simulink model "mVeh_fun_tbm"  (R2023b)
settings: Solver=FixedStepDiscrete  StartTime=0.0  StopTime=Parm_cnv_simulink_stopTime  FixedStep=Const_cnv_fundmt_stepSize  RelTol=1e-3  EnableMultiTasking=on
InitFcn:
  | preLoadFun
undefined symbols (not defined in the file or in its folder): Calib_pirelle_presSnr_x8, Calib_roadTriger_x6, Calib_tbm_brkBts_x8, Calib_tbm_ctr_x8, Calib_tbm_sensor_x4, Calib_tbm_strDistb_x8, Calib_tbm_supCtr_x8, CtrSet_tbm_enab_x8, IO397, Parm_tbmVeh_sig_max_numInvalid, Parm_tbmVeh_sig_tolerate_numInvalid
libraries: canmsglib x34, speedgoatlib_IO691 x19, MyLibrary x5, libtb_gen_canMsgCntr x5, speedgoatlib_fpga_analog_io x1, simulink x1, speedgoatlib_fpga x1, lib_decmp_CtrSet_tbm_enab_x8 x1, lib_decmp_Calib_tbm_brkPreTriger_x6 x1, lib_decmp_Calib_tbm_sensor_x4 x1
(part 3 of 3)

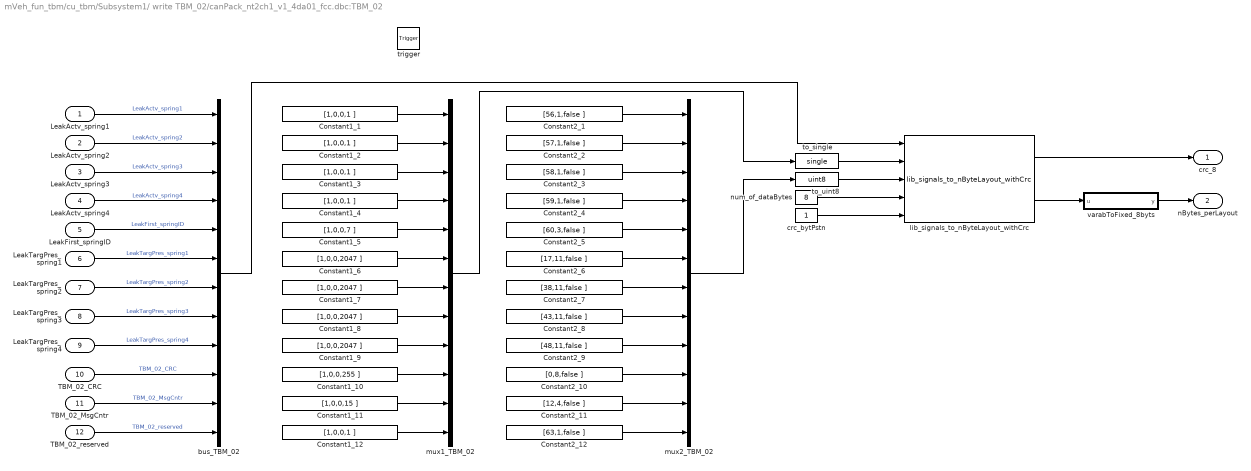
== system mVeh_fun_tbm/cu_tbm/Subsystem1/ write TBM_02/canPack_nt2ch1_v1_4da01_fcc.dbc:TBM_02 ==
  LeakActv_spring1 : Inport
  LeakActv_spring2 : Inport  Port=2
  LeakActv_spring3 : Inport  Port=3
  LeakActv_spring4 : Inport  Port=4
  LeakFirst_springID : Inport  Port=5
  LeakTargPres_spring1 : Inport  Port=6
  LeakTargPres_spring2 : Inport  Port=7
  LeakTargPres_spring3 : Inport  Port=8
  LeakTargPres_spring4 : Inport  Port=9
  TBM_02_CRC : Inport  Port=10
  TBM_02_MsgCntr : Inport  Port=11
  TBM_02_reserved : Inport  Port=12
  trigger : TriggerPort  TriggerType=either  VariantControl=Variant  PortDimensions=1
  Constant1_{1..4,12} (5 alike) : Constant  Value=[1,0,0,1 ]  SampleTime=-1
  Constant1_10 : Constant  Value=[1,0,0,255 ]  SampleTime=-1
  Constant1_11 : Constant  Value=[1,0,0,15 ]  SampleTime=-1
  Constant1_5 : Constant  Value=[1,0,0,7 ]  SampleTime=-1
  Constant1_{6..9} (4 alike) : Constant  Value=[1,0,0,2047 ]  SampleTime=-1
  Constant2_1 : Constant  Value=[56,1,false ]  SampleTime=-1
  Constant2_10 : Constant  Value=[0,8,false ]  SampleTime=-1
  Constant2_11 : Constant  Value=[12,4,false ]  SampleTime=-1
  Constant2_12 : Constant  Value=[63,1,false ]  SampleTime=-1
  Constant2_2 : Constant  Value=[57,1,false ]  SampleTime=-1
  Constant2_3 : Constant  Value=[58,1,false ]  SampleTime=-1
  Constant2_4 : Constant  Value=[59,1,false ]  SampleTime=-1
  Constant2_5 : Constant  Value=[60,3,false ]  SampleTime=-1
  Constant2_6 : Constant  Value=[17,11,false ]  SampleTime=-1
  Constant2_7 : Constant  Value=[38,11,false ]  SampleTime=-1
  Constant2_8 : Constant  Value=[43,11,false ]  SampleTime=-1
  Constant2_9 : Constant  Value=[48,11,false ]  SampleTime=-1
  bus_TBM_02 : BusCreator  Inputs=12
  crc_bytPstn : Constant  OutDataTypeStr=uint8  SampleTime=-1
  lib_signals_to_nByteLayout_withCrc : MyLibrary/lib_signals_to_nByteLayout_withCrc  SystemSampleTime=-1  VariantActivationTime=update diagram  AllowFlexibleInterface=on  Latency=0  AutoFrameSizeCalculation=off
  mux1_TBM_02 : Mux  Inputs=12
  mux2_TBM_02 : Mux  Inputs=12
  num_of_dataBytes : Constant  Value=8  OutDataTypeStr=uint8  SampleTime=-1
  to_single : DataTypeConversion  OutDataTypeStr=single  SaturateOnIntegerOverflow=off  RndMeth=Floor
  to_uint8 : DataTypeConversion  OutDataTypeStr=uint8  SaturateOnIntegerOverflow=off  RndMeth=Floor
  varabToFixed_8byts : MATLAB Function  TreatAsAtomicUnit=on
  crc_8 : Outport
  nBytes_perLayout : Outport  Port=2
  wires:
  LeakActv_spring1/1 -> bus_TBM_02/1  "LeakActv_spring1"
  LeakActv_spring2/1 -> bus_TBM_02/2  "LeakActv_spring2"
  LeakActv_spring3/1 -> bus_TBM_02/3  "LeakActv_spring3"
  LeakActv_spring4/1 -> bus_TBM_02/4  "LeakActv_spring4"
  LeakFirst_springID/1 -> bus_TBM_02/5  "LeakFirst_springID"
  LeakTargPres_spring1/1 -> bus_TBM_02/6  "LeakTargPres_spring1"
  LeakTargPres_spring2/1 -> bus_TBM_02/7  "LeakTargPres_spring2"
  LeakTargPres_spring3/1 -> bus_TBM_02/8  "LeakTargPres_spring3"
  LeakTargPres_spring4/1 -> bus_TBM_02/9  "LeakTargPres_spring4"
  TBM_02_CRC/1 -> bus_TBM_02/10  "TBM_02_CRC"
  TBM_02_MsgCntr/1 -> bus_TBM_02/11  "TBM_02_MsgCntr"
  TBM_02_reserved/1 -> bus_TBM_02/12  "TBM_02_reserved"
  Constant1_1/1 -> mux1_TBM_02/1
  Constant2_1/1 -> mux2_TBM_02/1
  Constant1_2/1 -> mux1_TBM_02/2
  Constant2_2/1 -> mux2_TBM_02/2
  Constant1_3/1 -> mux1_TBM_02/3
  Constant2_3/1 -> mux2_TBM_02/3
  Constant1_4/1 -> mux1_TBM_02/4
  Constant2_4/1 -> mux2_TBM_02/4
  Constant1_5/1 -> mux1_TBM_02/5
  Constant2_5/1 -> mux2_TBM_02/5
  Constant1_6/1 -> mux1_TBM_02/6
  Constant2_6/1 -> mux2_TBM_02/6
  Constant1_7/1 -> mux1_TBM_02/7
  Constant2_7/1 -> mux2_TBM_02/7
  Constant1_8/1 -> mux1_TBM_02/8
  Constant2_8/1 -> mux2_TBM_02/8
  Constant1_9/1 -> mux1_TBM_02/9
  Constant2_9/1 -> mux2_TBM_02/9
  Constant1_10/1 -> mux1_TBM_02/10
  Constant2_10/1 -> mux2_TBM_02/10
  Constant1_11/1 -> mux1_TBM_02/11
  Constant2_11/1 -> mux2_TBM_02/11
  Constant1_12/1 -> mux1_TBM_02/12
  Constant2_12/1 -> mux2_TBM_02/12
  bus_TBM_02/1 -> lib_signals_to_nByteLayout_withCrc/1
  mux1_TBM_02/1 -> to_single/1
  to_single/1 -> lib_signals_to_nByteLayout_withCrc/2
  mux2_TBM_02/1 -> to_uint8/1
  to_uint8/1 -> lib_signals_to_nByteLayout_withCrc/3
  lib_signals_to_nByteLayout_withCrc/1 -> crc_8/1
  num_of_dataBytes/1 -> lib_signals_to_nByteLayout_withCrc/4
  lib_signals_to_nByteLayout_withCrc/2 -> varabToFixed_8byts/1(u)
  varabToFixed_8byts/1(y) -> nBytes_perLayout/1
  crc_bytPstn/1 -> lib_signals_to_nByteLayout_withCrc/5

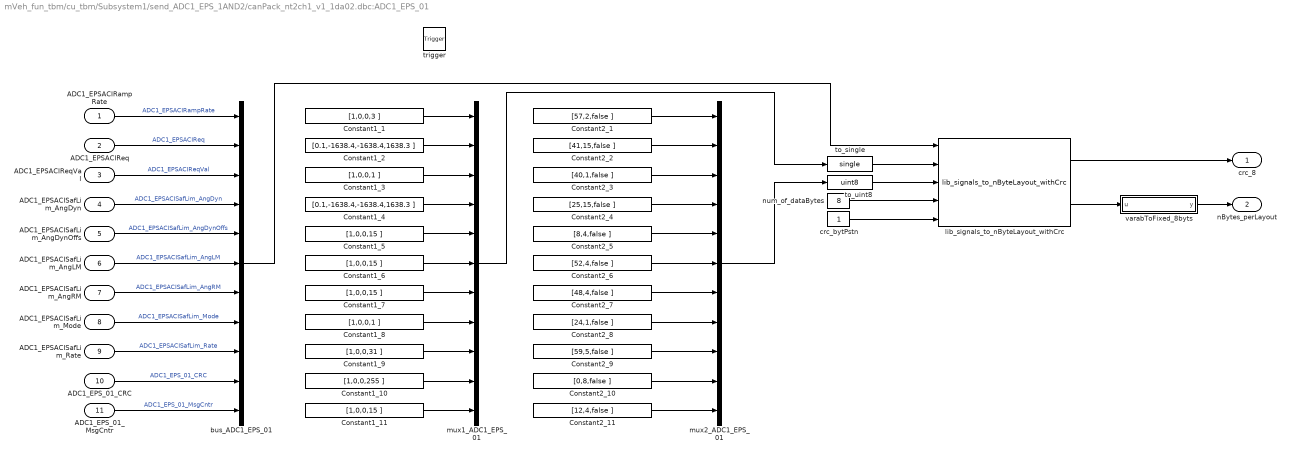
== system mVeh_fun_tbm/cu_tbm/Subsystem1/send_ADC1_EPS_1AND2/canPack_nt2ch1_v1_1da02.dbc:ADC1_EPS_01 ==
  ADC1_EPSACIRampRate : Inport
  ADC1_EPSACIReq : Inport  Port=2
  ADC1_EPSACIReqVal : Inport  Port=3
  ADC1_EPSACISafLim_AngDyn : Inport  Port=4
  ADC1_EPSACISafLim_AngDynOffs : Inport  Port=5
  ADC1_EPSACISafLim_AngLM : Inport  Port=6
  ADC1_EPSACISafLim_AngRM : Inport  Port=7
  ADC1_EPSACISafLim_Mode : Inport  Port=8
  ADC1_EPSACISafLim_Rate : Inport  Port=9
  ADC1_EPS_01_CRC : Inport  Port=10
  ADC1_EPS_01_MsgCntr : Inport  Port=11
  trigger : TriggerPort  TriggerType=either  VariantControl=Variant  PortDimensions=1
  Constant1_1 : Constant  Value=[1,0,0,3 ]  SampleTime=-1
  Constant1_10 : Constant  Value=[1,0,0,255 ]  SampleTime=-1
  Constant1_{5..7,11} (4 alike) : Constant  Value=[1,0,0,15 ]  SampleTime=-1
  Constant1_2 : Constant  Value=[0.1,-1638.4,-1638.4,1638.3 ]  SampleTime=-1
  Constant1_3 : Constant  Value=[1,0,0,1 ]  SampleTime=-1
  Constant1_4 : Constant  Value=[0.1,-1638.4,-1638.4,1638.3 ]  SampleTime=-1
  Constant1_8 : Constant  Value=[1,0,0,1 ]  SampleTime=-1
  Constant1_9 : Constant  Value=[1,0,0,31 ]  SampleTime=-1
  Constant2_1 : Constant  Value=[57,2,false ]  SampleTime=-1
  Constant2_10 : Constant  Value=[0,8,false ]  SampleTime=-1
  Constant2_11 : Constant  Value=[12,4,false ]  SampleTime=-1
  Constant2_2 : Constant  Value=[41,15,false ]  SampleTime=-1
  Constant2_3 : Constant  Value=[40,1,false ]  SampleTime=-1
  Constant2_4 : Constant  Value=[25,15,false ]  SampleTime=-1
  Constant2_5 : Constant  Value=[8,4,false ]  SampleTime=-1
  Constant2_6 : Constant  Value=[52,4,false ]  SampleTime=-1
  Constant2_7 : Constant  Value=[48,4,false ]  SampleTime=-1
  Constant2_8 : Constant  Value=[24,1,false ]  SampleTime=-1
  Constant2_9 : Constant  Value=[59,5,false ]  SampleTime=-1
  bus_ADC1_EPS_01 : BusCreator  Inputs=11
  crc_bytPstn : Constant  OutDataTypeStr=uint8  SampleTime=-1
  lib_signals_to_nByteLayout_withCrc : MyLibrary/lib_signals_to_nByteLayout_withCrc  SystemSampleTime=-1  VariantActivationTime=update diagram  AllowFlexibleInterface=on  Latency=0  AutoFrameSizeCalculation=off
  mux1_ADC1_EPS_01 : Mux  Inputs=11
  mux2_ADC1_EPS_01 : Mux  Inputs=11
  num_of_dataBytes : Constant  Value=8  OutDataTypeStr=uint8  SampleTime=-1
  to_single : DataTypeConversion  OutDataTypeStr=single  SaturateOnIntegerOverflow=off  RndMeth=Floor
  to_uint8 : DataTypeConversion  OutDataTypeStr=uint8  SaturateOnIntegerOverflow=off  RndMeth=Floor
  varabToFixed_8byts : MATLAB Function  TreatAsAtomicUnit=on
  crc_8 : Outport
  nBytes_perLayout : Outport  Port=2
  wires:
  ADC1_EPSACIRampRate/1 -> bus_ADC1_EPS_01/1  "ADC1_EPSACIRampRate"
  ADC1_EPSACIReq/1 -> bus_ADC1_EPS_01/2  "ADC1_EPSACIReq"
  ADC1_EPSACIReqVal/1 -> bus_ADC1_EPS_01/3  "ADC1_EPSACIReqVal"
  ADC1_EPSACISafLim_AngDyn/1 -> bus_ADC1_EPS_01/4  "ADC1_EPSACISafLim_AngDyn"
  ADC1_EPSACISafLim_AngDynOffs/1 -> bus_ADC1_EPS_01/5  "ADC1_EPSACISafLim_AngDynOffs"
  ADC1_EPSACISafLim_AngLM/1 -> bus_ADC1_EPS_01/6  "ADC1_EPSACISafLim_AngLM"
  ADC1_EPSACISafLim_AngRM/1 -> bus_ADC1_EPS_01/7  "ADC1_EPSACISafLim_AngRM"
  ADC1_EPSACISafLim_Mode/1 -> bus_ADC1_EPS_01/8  "ADC1_EPSACISafLim_Mode"
  ADC1_EPSACISafLim_Rate/1 -> bus_ADC1_EPS_01/9  "ADC1_EPSACISafLim_Rate"
  ADC1_EPS_01_CRC/1 -> bus_ADC1_EPS_01/10  "ADC1_EPS_01_CRC"
  ADC1_EPS_01_MsgCntr/1 -> bus_ADC1_EPS_01/11  "ADC1_EPS_01_MsgCntr"
  Constant1_1/1 -> mux1_ADC1_EPS_01/1
  Constant2_1/1 -> mux2_ADC1_EPS_01/1
  Constant1_2/1 -> mux1_ADC1_EPS_01/2
  Constant2_2/1 -> mux2_ADC1_EPS_01/2
  Constant1_3/1 -> mux1_ADC1_EPS_01/3
  Constant2_3/1 -> mux2_ADC1_EPS_01/3
  Constant1_4/1 -> mux1_ADC1_EPS_01/4
  Constant2_4/1 -> mux2_ADC1_EPS_01/4
  Constant1_5/1 -> mux1_ADC1_EPS_01/5
  Constant2_5/1 -> mux2_ADC1_EPS_01/5
  Constant1_6/1 -> mux1_ADC1_EPS_01/6
  Constant2_6/1 -> mux2_ADC1_EPS_01/6
  Constant1_7/1 -> mux1_ADC1_EPS_01/7
  Constant2_7/1 -> mux2_ADC1_EPS_01/7
  Constant1_8/1 -> mux1_ADC1_EPS_01/8
  Constant2_8/1 -> mux2_ADC1_EPS_01/8
  Constant1_9/1 -> mux1_ADC1_EPS_01/9
  Constant2_9/1 -> mux2_ADC1_EPS_01/9
  Constant1_10/1 -> mux1_ADC1_EPS_01/10
  Constant2_10/1 -> mux2_ADC1_EPS_01/10
  Constant1_11/1 -> mux1_ADC1_EPS_01/11
  Constant2_11/1 -> mux2_ADC1_EPS_01/11
  bus_ADC1_EPS_01/1 -> lib_signals_to_nByteLayout_withCrc/1
  mux1_ADC1_EPS_01/1 -> to_single/1
  to_single/1 -> lib_signals_to_nByteLayout_withCrc/2
  mux2_ADC1_EPS_01/1 -> to_uint8/1
  to_uint8/1 -> lib_signals_to_nByteLayout_withCrc/3
  lib_signals_to_nByteLayout_withCrc/1 -> crc_8/1
  num_of_dataBytes/1 -> lib_signals_to_nByteLayout_withCrc/4
  lib_signals_to_nByteLayout_withCrc/2 -> varabToFixed_8byts/1(u)
  varabToFixed_8byts/1(y) -> nBytes_perLayout/1
  crc_bytPstn/1 -> lib_signals_to_nByteLayout_withCrc/5

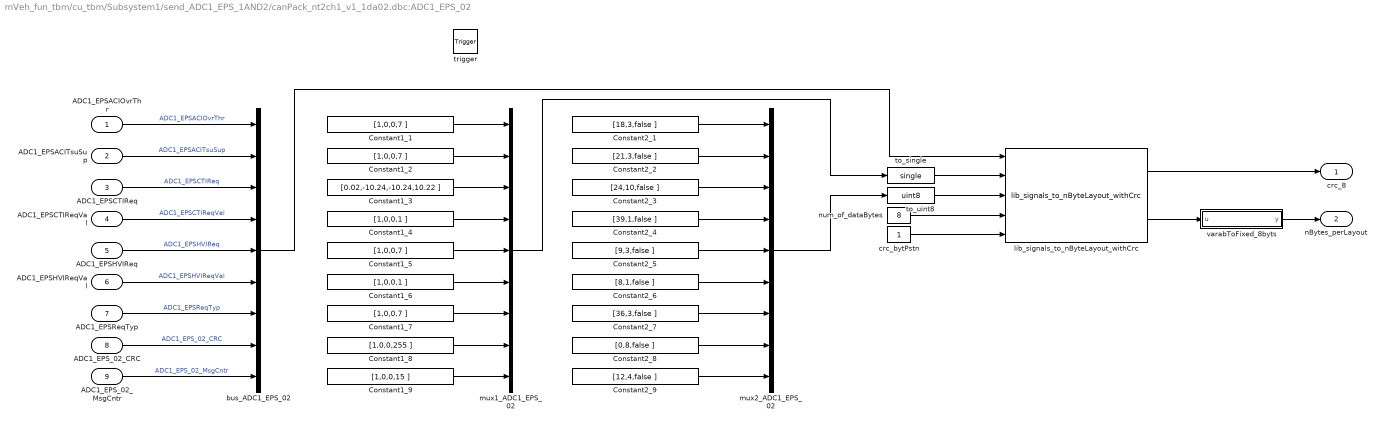
== system mVeh_fun_tbm/cu_tbm/Subsystem1/send_ADC1_EPS_1AND2/canPack_nt2ch1_v1_1da02.dbc:ADC1_EPS_02 ==
  ADC1_EPSACIOvrThr : Inport
  ADC1_EPSACITsuSup : Inport  Port=2
  ADC1_EPSCTIReq : Inport  Port=3
  ADC1_EPSCTIReqVal : Inport  Port=4
  ADC1_EPSHVIReq : Inport  Port=5
  ADC1_EPSHVIReqVal : Inport  Port=6
  ADC1_EPSReqTyp : Inport  Port=7
  ADC1_EPS_02_CRC : Inport  Port=8
  ADC1_EPS_02_MsgCntr : Inport  Port=9
  trigger : TriggerPort  TriggerType=either  VariantControl=Variant  PortDimensions=1
  Constant1_{1..2,5,7} (4 alike) : Constant  Value=[1,0,0,7 ]  SampleTime=-1
  Constant1_3 : Constant  Value=[0.02,-10.24,-10.24,10.22 ]  SampleTime=-1
  Constant1_4 : Constant  Value=[1,0,0,1 ]  SampleTime=-1
  Constant1_6 : Constant  Value=[1,0,0,1 ]  SampleTime=-1
  Constant1_8 : Constant  Value=[1,0,0,255 ]  SampleTime=-1
  Constant1_9 : Constant  Value=[1,0,0,15 ]  SampleTime=-1
  Constant2_1 : Constant  Value=[18,3,false ]  SampleTime=-1
  Constant2_2 : Constant  Value=[21,3,false ]  SampleTime=-1
  Constant2_3 : Constant  Value=[24,10,false ]  SampleTime=-1
  Constant2_4 : Constant  Value=[39,1,false ]  SampleTime=-1
  Constant2_5 : Constant  Value=[9,3,false ]  SampleTime=-1
  Constant2_6 : Constant  Value=[8,1,false ]  SampleTime=-1
  Constant2_7 : Constant  Value=[36,3,false ]  SampleTime=-1
  Constant2_8 : Constant  Value=[0,8,false ]  SampleTime=-1
  Constant2_9 : Constant  Value=[12,4,false ]  SampleTime=-1
  bus_ADC1_EPS_02 : BusCreator  Inputs=9
  crc_bytPstn : Constant  OutDataTypeStr=uint8  SampleTime=-1
  lib_signals_to_nByteLayout_withCrc : MyLibrary/lib_signals_to_nByteLayout_withCrc  SystemSampleTime=-1  VariantActivationTime=update diagram  AllowFlexibleInterface=on  Latency=0  AutoFrameSizeCalculation=off
  mux1_ADC1_EPS_02 : Mux  Inputs=9
  mux2_ADC1_EPS_02 : Mux  Inputs=9
  num_of_dataBytes : Constant  Value=8  OutDataTypeStr=uint8  SampleTime=-1
  to_single : DataTypeConversion  OutDataTypeStr=single  SaturateOnIntegerOverflow=off  RndMeth=Floor
  to_uint8 : DataTypeConversion  OutDataTypeStr=uint8  SaturateOnIntegerOverflow=off  RndMeth=Floor
  varabToFixed_8byts : MATLAB Function  TreatAsAtomicUnit=on
  crc_8 : Outport
  nBytes_perLayout : Outport  Port=2
  wires:
  ADC1_EPSACIOvrThr/1 -> bus_ADC1_EPS_02/1  "ADC1_EPSACIOvrThr"
  ADC1_EPSACITsuSup/1 -> bus_ADC1_EPS_02/2  "ADC1_EPSACITsuSup"
  ADC1_EPSCTIReq/1 -> bus_ADC1_EPS_02/3  "ADC1_EPSCTIReq"
  ADC1_EPSCTIReqVal/1 -> bus_ADC1_EPS_02/4  "ADC1_EPSCTIReqVal"
  ADC1_EPSHVIReq/1 -> bus_ADC1_EPS_02/5  "ADC1_EPSHVIReq"
  ADC1_EPSHVIReqVal/1 -> bus_ADC1_EPS_02/6  "ADC1_EPSHVIReqVal"
  ADC1_EPSReqTyp/1 -> bus_ADC1_EPS_02/7  "ADC1_EPSReqTyp"
  ADC1_EPS_02_CRC/1 -> bus_ADC1_EPS_02/8  "ADC1_EPS_02_CRC"
  ADC1_EPS_02_MsgCntr/1 -> bus_ADC1_EPS_02/9  "ADC1_EPS_02_MsgCntr"
  Constant1_1/1 -> mux1_ADC1_EPS_02/1
  Constant2_1/1 -> mux2_ADC1_EPS_02/1
  Constant1_2/1 -> mux1_ADC1_EPS_02/2
  Constant2_2/1 -> mux2_ADC1_EPS_02/2
  Constant1_3/1 -> mux1_ADC1_EPS_02/3
  Constant2_3/1 -> mux2_ADC1_EPS_02/3
  Constant1_4/1 -> mux1_ADC1_EPS_02/4
  Constant2_4/1 -> mux2_ADC1_EPS_02/4
  Constant1_5/1 -> mux1_ADC1_EPS_02/5
  Constant2_5/1 -> mux2_ADC1_EPS_02/5
  Constant1_6/1 -> mux1_ADC1_EPS_02/6
  Constant2_6/1 -> mux2_ADC1_EPS_02/6
  Constant1_7/1 -> mux1_ADC1_EPS_02/7
  Constant2_7/1 -> mux2_ADC1_EPS_02/7
  Constant1_8/1 -> mux1_ADC1_EPS_02/8
  Constant2_8/1 -> mux2_ADC1_EPS_02/8
  Constant1_9/1 -> mux1_ADC1_EPS_02/9
  Constant2_9/1 -> mux2_ADC1_EPS_02/9
  bus_ADC1_EPS_02/1 -> lib_signals_to_nByteLayout_withCrc/1
  mux1_ADC1_EPS_02/1 -> to_single/1
  to_single/1 -> lib_signals_to_nByteLayout_withCrc/2
  mux2_ADC1_EPS_02/1 -> to_uint8/1
  to_uint8/1 -> lib_signals_to_nByteLayout_withCrc/3
  lib_signals_to_nByteLayout_withCrc/1 -> crc_8/1
  num_of_dataBytes/1 -> lib_signals_to_nByteLayout_withCrc/4
  lib_signals_to_nByteLayout_withCrc/2 -> varabToFixed_8byts/1(u)
  varabToFixed_8byts/1(y) -> nBytes_perLayout/1
  crc_bytPstn/1 -> lib_signals_to_nByteLayout_withCrc/5

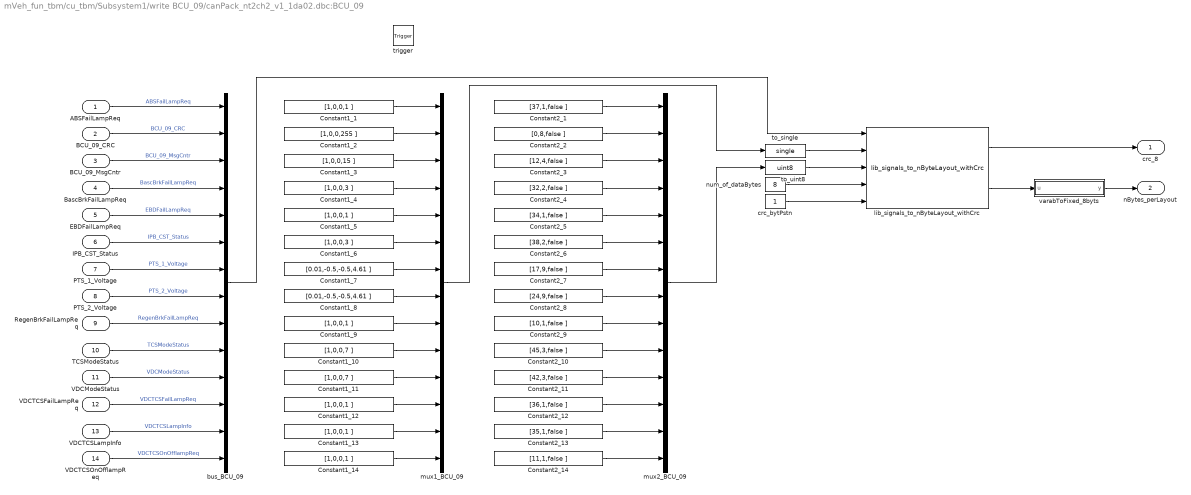
== system mVeh_fun_tbm/cu_tbm/Subsystem1/write BCU_09/canPack_nt2ch2_v1_1da02.dbc:BCU_09 ==
  ABSFailLampReq : Inport
  BCU_09_CRC : Inport  Port=2
  BCU_09_MsgCntr : Inport  Port=3
  BascBrkFailLampReq : Inport  Port=4
  EBDFailLampReq : Inport  Port=5
  IPB_CST_Status : Inport  Port=6
  PTS_1_Voltage : Inport  Port=7
  PTS_2_Voltage : Inport  Port=8
  RegenBrkFailLampReq : Inport  Port=9
  TCSModeStatus : Inport  Port=10
  VDCModeStatus : Inport  Port=11
  VDCTCSFailLampReq : Inport  Port=12
  VDCTCSLampInfo : Inport  Port=13
  VDCTCSOnOfflampReq : Inport  Port=14
  trigger : TriggerPort  TriggerType=either  VariantControl=Variant  PortDimensions=1
  Constant1_{1,5,9,12..14} (6 alike) : Constant  Value=[1,0,0,1 ]  SampleTime=-1
  Constant1_10 : Constant  Value=[1,0,0,7 ]  SampleTime=-1
  Constant1_11 : Constant  Value=[1,0,0,7 ]  SampleTime=-1
  Constant1_2 : Constant  Value=[1,0,0,255 ]  SampleTime=-1
  Constant1_3 : Constant  Value=[1,0,0,15 ]  SampleTime=-1
  Constant1_4 : Constant  Value=[1,0,0,3 ]  SampleTime=-1
  Constant1_6 : Constant  Value=[1,0,0,3 ]  SampleTime=-1
  Constant1_7 : Constant  Value=[0.01,-0.5,-0.5,4.61 ]  SampleTime=-1
  Constant1_8 : Constant  Value=[0.01,-0.5,-0.5,4.61 ]  SampleTime=-1
  Constant2_1 : Constant  Value=[37,1,false ]  SampleTime=-1
  Constant2_10 : Constant  Value=[45,3,false ]  SampleTime=-1
  Constant2_11 : Constant  Value=[42,3,false ]  SampleTime=-1
  Constant2_12 : Constant  Value=[36,1,false ]  SampleTime=-1
  Constant2_13 : Constant  Value=[35,1,false ]  SampleTime=-1
  Constant2_14 : Constant  Value=[11,1,false ]  SampleTime=-1
  Constant2_2 : Constant  Value=[0,8,false ]  SampleTime=-1
  Constant2_3 : Constant  Value=[12,4,false ]  SampleTime=-1
  Constant2_4 : Constant  Value=[32,2,false ]  SampleTime=-1
  Constant2_5 : Constant  Value=[34,1,false ]  SampleTime=-1
  Constant2_6 : Constant  Value=[38,2,false ]  SampleTime=-1
  Constant2_7 : Constant  Value=[17,9,false ]  SampleTime=-1
  Constant2_8 : Constant  Value=[24,9,false ]  SampleTime=-1
  Constant2_9 : Constant  Value=[10,1,false ]  SampleTime=-1
  bus_BCU_09 : BusCreator  Inputs=14
  crc_bytPstn : Constant  OutDataTypeStr=uint8  SampleTime=-1
  lib_signals_to_nByteLayout_withCrc : MyLibrary/lib_signals_to_nByteLayout_withCrc  SystemSampleTime=-1  VariantActivationTime=update diagram  AllowFlexibleInterface=on  Latency=0  AutoFrameSizeCalculation=off
  mux1_BCU_09 : Mux  Inputs=14
  mux2_BCU_09 : Mux  Inputs=14
  num_of_dataBytes : Constant  Value=8  OutDataTypeStr=uint8  SampleTime=-1
  to_single : DataTypeConversion  OutDataTypeStr=single  SaturateOnIntegerOverflow=off  RndMeth=Floor
  to_uint8 : DataTypeConversion  OutDataTypeStr=uint8  SaturateOnIntegerOverflow=off  RndMeth=Floor
  varabToFixed_8byts : MATLAB Function  TreatAsAtomicUnit=on
  crc_8 : Outport
  nBytes_perLayout : Outport  Port=2
  wires:
  ABSFailLampReq/1 -> bus_BCU_09/1  "ABSFailLampReq"
  BCU_09_CRC/1 -> bus_BCU_09/2  "BCU_09_CRC"
  BCU_09_MsgCntr/1 -> bus_BCU_09/3  "BCU_09_MsgCntr"
  BascBrkFailLampReq/1 -> bus_BCU_09/4  "BascBrkFailLampReq"
  EBDFailLampReq/1 -> bus_BCU_09/5  "EBDFailLampReq"
  IPB_CST_Status/1 -> bus_BCU_09/6  "IPB_CST_Status"
  PTS_1_Voltage/1 -> bus_BCU_09/7  "PTS_1_Voltage"
  PTS_2_Voltage/1 -> bus_BCU_09/8  "PTS_2_Voltage"
  RegenBrkFailLampReq/1 -> bus_BCU_09/9  "RegenBrkFailLampReq"
  TCSModeStatus/1 -> bus_BCU_09/10  "TCSModeStatus"
  VDCModeStatus/1 -> bus_BCU_09/11  "VDCModeStatus"
  VDCTCSFailLampReq/1 -> bus_BCU_09/12  "VDCTCSFailLampReq"
  VDCTCSLampInfo/1 -> bus_BCU_09/13  "VDCTCSLampInfo"
  VDCTCSOnOfflampReq/1 -> bus_BCU_09/14  "VDCTCSOnOfflampReq"
  Constant1_1/1 -> mux1_BCU_09/1
  Constant2_1/1 -> mux2_BCU_09/1
  Constant1_2/1 -> mux1_BCU_09/2
  Constant2_2/1 -> mux2_BCU_09/2
  Constant1_3/1 -> mux1_BCU_09/3
  Constant2_3/1 -> mux2_BCU_09/3
  Constant1_4/1 -> mux1_BCU_09/4
  Constant2_4/1 -> mux2_BCU_09/4
  Constant1_5/1 -> mux1_BCU_09/5
  Constant2_5/1 -> mux2_BCU_09/5
  Constant1_6/1 -> mux1_BCU_09/6
  Constant2_6/1 -> mux2_BCU_09/6
  Constant1_7/1 -> mux1_BCU_09/7
  Constant2_7/1 -> mux2_BCU_09/7
  Constant1_8/1 -> mux1_BCU_09/8
  Constant2_8/1 -> mux2_BCU_09/8
  Constant1_9/1 -> mux1_BCU_09/9
  Constant2_9/1 -> mux2_BCU_09/9
  Constant1_10/1 -> mux1_BCU_09/10
  Constant2_10/1 -> mux2_BCU_09/10
  Constant1_11/1 -> mux1_BCU_09/11
  Constant2_11/1 -> mux2_BCU_09/11
  Constant1_12/1 -> mux1_BCU_09/12
  Constant2_12/1 -> mux2_BCU_09/12
  Constant1_13/1 -> mux1_BCU_09/13
  Constant2_13/1 -> mux2_BCU_09/13
  Constant1_14/1 -> mux1_BCU_09/14
  Constant2_14/1 -> mux2_BCU_09/14
  bus_BCU_09/1 -> lib_signals_to_nByteLayout_withCrc/1
  mux1_BCU_09/1 -> to_single/1
  to_single/1 -> lib_signals_to_nByteLayout_withCrc/2
  mux2_BCU_09/1 -> to_uint8/1
  to_uint8/1 -> lib_signals_to_nByteLayout_withCrc/3
  lib_signals_to_nByteLayout_withCrc/1 -> crc_8/1
  num_of_dataBytes/1 -> lib_signals_to_nByteLayout_withCrc/4
  lib_signals_to_nByteLayout_withCrc/2 -> varabToFixed_8byts/1(u)
  varabToFixed_8byts/1(y) -> nBytes_perLayout/1
  crc_bytPstn/1 -> lib_signals_to_nByteLayout_withCrc/5

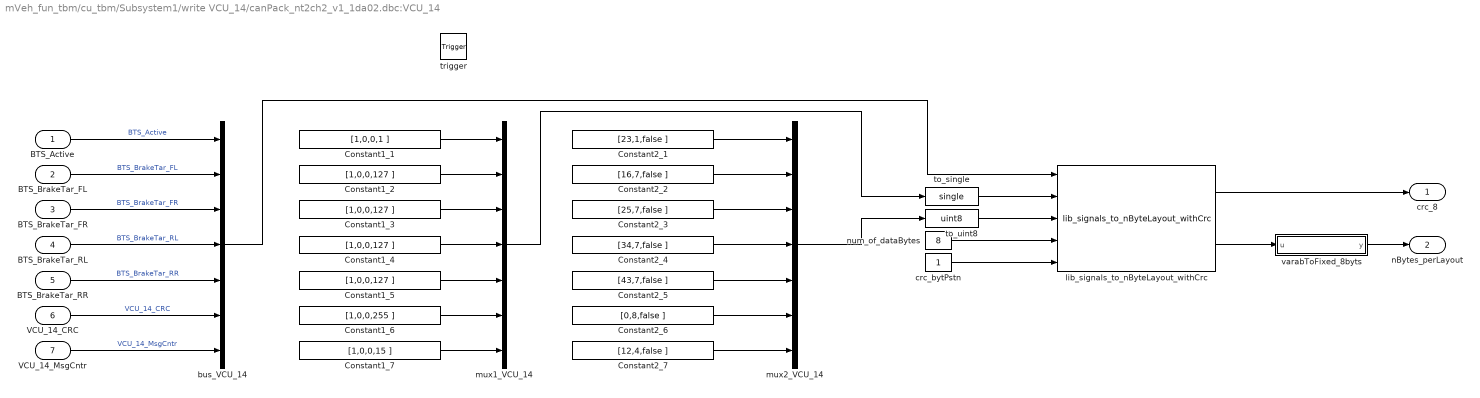
== system mVeh_fun_tbm/cu_tbm/Subsystem1/write VCU_14/canPack_nt2ch2_v1_1da02.dbc:VCU_14 ==
  BTS_Active : Inport
  BTS_BrakeTar_FL : Inport  Port=2
  BTS_BrakeTar_FR : Inport  Port=3
  BTS_BrakeTar_RL : Inport  Port=4
  BTS_BrakeTar_RR : Inport  Port=5
  VCU_14_CRC : Inport  Port=6
  VCU_14_MsgCntr : Inport  Port=7
  trigger : TriggerPort  TriggerType=either  VariantControl=Variant  PortDimensions=1
  Constant1_1 : Constant  Value=[1,0,0,1 ]  SampleTime=-1
  Constant1_{2..5} (4 alike) : Constant  Value=[1,0,0,127 ]  SampleTime=-1
  Constant1_6 : Constant  Value=[1,0,0,255 ]  SampleTime=-1
  Constant1_7 : Constant  Value=[1,0,0,15 ]  SampleTime=-1
  Constant2_1 : Constant  Value=[23,1,false ]  SampleTime=-1
  Constant2_2 : Constant  Value=[16,7,false ]  SampleTime=-1
  Constant2_3 : Constant  Value=[25,7,false ]  SampleTime=-1
  Constant2_4 : Constant  Value=[34,7,false ]  SampleTime=-1
  Constant2_5 : Constant  Value=[43,7,false ]  SampleTime=-1
  Constant2_6 : Constant  Value=[0,8,false ]  SampleTime=-1
  Constant2_7 : Constant  Value=[12,4,false ]  SampleTime=-1
  bus_VCU_14 : BusCreator  Inputs=7
  crc_bytPstn : Constant  OutDataTypeStr=uint8  SampleTime=-1
  lib_signals_to_nByteLayout_withCrc : MyLibrary/lib_signals_to_nByteLayout_withCrc  SystemSampleTime=-1  VariantActivationTime=update diagram  AllowFlexibleInterface=on  Latency=0  AutoFrameSizeCalculation=off
  mux1_VCU_14 : Mux  Inputs=7
  mux2_VCU_14 : Mux  Inputs=7
  num_of_dataBytes : Constant  Value=8  OutDataTypeStr=uint8  SampleTime=-1
  to_single : DataTypeConversion  OutDataTypeStr=single  SaturateOnIntegerOverflow=off  RndMeth=Floor
  to_uint8 : DataTypeConversion  OutDataTypeStr=uint8  SaturateOnIntegerOverflow=off  RndMeth=Floor
  varabToFixed_8byts : MATLAB Function  TreatAsAtomicUnit=on
  crc_8 : Outport
  nBytes_perLayout : Outport  Port=2
  wires:
  BTS_Active/1 -> bus_VCU_14/1  "BTS_Active"
  BTS_BrakeTar_FL/1 -> bus_VCU_14/2  "BTS_BrakeTar_FL"
  BTS_BrakeTar_FR/1 -> bus_VCU_14/3  "BTS_BrakeTar_FR"
  BTS_BrakeTar_RL/1 -> bus_VCU_14/4  "BTS_BrakeTar_RL"
  BTS_BrakeTar_RR/1 -> bus_VCU_14/5  "BTS_BrakeTar_RR"
  VCU_14_CRC/1 -> bus_VCU_14/6  "VCU_14_CRC"
  VCU_14_MsgCntr/1 -> bus_VCU_14/7  "VCU_14_MsgCntr"
  Constant1_1/1 -> mux1_VCU_14/1
  Constant2_1/1 -> mux2_VCU_14/1
  Constant1_2/1 -> mux1_VCU_14/2
  Constant2_2/1 -> mux2_VCU_14/2
  Constant1_3/1 -> mux1_VCU_14/3
  Constant2_3/1 -> mux2_VCU_14/3
  Constant1_4/1 -> mux1_VCU_14/4
  Constant2_4/1 -> mux2_VCU_14/4
  Constant1_5/1 -> mux1_VCU_14/5
  Constant2_5/1 -> mux2_VCU_14/5
  Constant1_6/1 -> mux1_VCU_14/6
  Constant2_6/1 -> mux2_VCU_14/6
  Constant1_7/1 -> mux1_VCU_14/7
  Constant2_7/1 -> mux2_VCU_14/7
  bus_VCU_14/1 -> lib_signals_to_nByteLayout_withCrc/1
  mux1_VCU_14/1 -> to_single/1
  to_single/1 -> lib_signals_to_nByteLayout_withCrc/2
  mux2_VCU_14/1 -> to_uint8/1
  to_uint8/1 -> lib_signals_to_nByteLayout_withCrc/3
  lib_signals_to_nByteLayout_withCrc/1 -> crc_8/1
  num_of_dataBytes/1 -> lib_signals_to_nByteLayout_withCrc/4
  lib_signals_to_nByteLayout_withCrc/2 -> varabToFixed_8byts/1(u)
  varabToFixed_8byts/1(y) -> nBytes_perLayout/1
  crc_bytPstn/1 -> lib_signals_to_nByteLayout_withCrc/5

== matlab function mVeh_fun_tbm/cu_tbm/Equation/MATLAB Function1 ==
  data: u input; y output
function y = fcn(u)

 y = 0.01 * u - 6.04;

== matlab function mVeh_fun_tbm/cu_tbm/MATLAB Function3 ==
  data: brkPdlTrvlCalSts input uint8; dr_isBrkg output boolean; brkPdlSts input uint8
function dr_isBrkg = fcn(brkPdlTrvlCalSts, brkPdlSts)


dr_isBrkg = false; 

if    ( brkPdlTrvlCalSts == uint8(1) ) ...      % 1 is brake pedal sensor calibrated
   && ( brkPdlSts == uint8(1)  )                % 1 is brkPdl pressed  

    dr_isBrkg = true; 


end

== matlab function mVeh_fun_tbm/cu_tbm/asm_canMsg/to_eps/MATLAB Function ==
  data: epsDist_enab input boolean; distbCtr_actv input boolean; epsReqType output uint8
function epsReqType = fcn (epsDist_enab, distbCtr_actv)

epsReqType = uint8(0);

if epsDist_enab && distbCtr_actv
    epsReqType = uint8(1);
end

== matlab function mVeh_fun_tbm/cu_tbm/Equation/MATLAB Function2 ==
  data: u input; y output
function y = fcn(u)

 y = 0.01 * u - 6.04;

== matlab function mVeh_fun_tbm/cu_tbm/Equation/MATLAB Function3 ==
  data: u input; y output
function y = fcn(u)

 y = 0.01 * u - 6.04;

== matlab function mVeh_fun_tbm/cu_tbm/asm_canMsg/to_bcu_bts/MATLAB Function ==
  data: btsCtr_actv output boolean; bts_enab input boolean; btsSimuDrBrk_actv input boolean; btsSimuDrBrk_pTgt_4w input single; bts_pTgt_4w output single size=4; tbmModfBrk_actv_4w input boolean size=4; tbmModfBrk_pTgt_4w input single size=4
function [btsCtr_actv, bts_pTgt_4w] = fcn (bts_enab, btsSimuDrBrk_actv, btsSimuDrBrk_pTgt_4w, tbmModfBrk_actv_4w, tbmModfBrk_pTgt_4w)

btsCtr_actv = false;
bts_pTgt_4w = [single(0); single(0); single(0); single(0)];

if bts_enab && btsSimuDrBrk_actv
    pTgt_4w = btsSimuDrBrk_pTgt_4w;
    btsCtr_actv = true;
    for w = 1:4
       if  tbmModfBrk_actv_4w(w) 
           
           pTgt_4w(w) = tbmModfBrk_pTgt_4w(w);
           
       end        
    end 
    bts_pTgt_4w = pTgt_4w; 
    
end

== stateflow chart mVeh_fun_tbm/cu_tbm/lib_gen_canMsgCntr1 ==
  state counter
  (default) -> counter : { count = 0}
  counter -> (junction 5) : {count = count+1;}
  (junction 5) -> counter [order 2]
  (junction 5) -> counter [order 1] : [count > 65534] {count = 0;}
  data: count output uint16
  events: event input RISING_EDGE_EVENT

== matlab function mVeh_fun_tbm/cu_tbm/Equation1/MATLAB Function ==
  data: u input; y output
function y = fcn(u)

 y = (u + 6.04) / 0.01;

== matlab function mVeh_fun_tbm/cu_tbm/Equation1/MATLAB Function1 ==
  data: u input; y output
function y = fcn(u)

 y = (u + 6.04) / 0.01;

== matlab function mVeh_fun_tbm/cu_tbm/Equation1/MATLAB Function2 ==
  data: u input; y output
function y = fcn(u)

 y = (u + 6.04) / 0.01;

== matlab function mVeh_fun_tbm/cu_tbm/Equation1/MATLAB Function3 ==
  data: u input; y output
function y = fcn(u)

 y = (u + 6.04) / 0.01;

== matlab function mVeh_fun_tbm/cu_tbm/spd_stsToValidity ==
  data: spd_valid output boolean; spd_status input uint8
function spd_valid  = fcn(spd_status)

if spd_status == 0 
    spd_valid = true; 
else
    spd_valid = false; 
end

== matlab function mVeh_fun_tbm/cu_tbm/Subsystem1/write BCU_09/canPack_nt2ch2_v1_1da02.dbc:BCU_09/varabToFixed_8byts ==
  data: u input uint8 size=8; y output uint8
function y = fcn(u)

fixed_size = 8;
y = uint8(zeros(fixed_size,1));

for i=1:fixed_size
    y(i) = u(i);
end

== matlab function mVeh_fun_tbm/cu_tbm/road_preTriger_brkByBts/MATLAB Function ==
  data: old_measure input double; measure_isNew output boolean; new_measure input double
function measure_isNew = fcn(old_measure, new_measure)

measure_isNew = false;

if old_measure ~= new_measure
    measure_isNew = true;
end

== stateflow chart mVeh_fun_tbm/cu_tbm/road_preTriger_brkByBts/sm_trigr_byHeitSnr ==
  state trigred
    en:
    st = 3;    trigred = true;
  state disregard
    en:
    st = 0;    trigred = false;
  state trigring
    en:
    st = 2;    trigred = false;
    state qualifed
      en:
      qalfd_numDat = qalfd_numDat +1;
    state unqualifed
      en:
      qalfd_numDat = qalfd_numDat -1;
    qualifed -> (junction 32)
    (junction 19) -> qualifed [order 1] : [      (measured_tgrGap < clb_gapMax) ...
        |   && (measured_tgrGap > clb_gapMin) ]
    (junction 32) -> (junction 19) : [measure_isNew]
    unqualifed -> (junction 32)
    (junction 19) -> unqualifed [order 2]
  state watch_for_trigr
    en:
    st = 1;    trigred = false;    qalfd_numDat = 0;
  (default) -> disregard
  trigred -> disregard : after(5, sec)
  trigring -> trigred [order 1] : [qalfd_numDat > clb_numDatMin ]
  disregard -> watch_for_trigr : [ load_trigr ]
  watch_for_trigr -> disregard [order 2] : [ ~load_trigr ]
  watch_for_trigr -> (junction 32) [order 1]
  trigring -> watch_for_trigr [order 2] : [qalfd_numDat <= 0 ]
  data: measure_isNew input boolean; measured_tgrGap input single size=1; load_trigr input boolean; clb_gapMax input single size=1; clb_gapMin input single size=1; trigred output boolean; clb_numDatMin input uint8 size=1; st output uint8; qalfd_numDat output uint8 size=1

== matlab function mVeh_fun_tbm/cu_tbm/tbm_sensor/perSnrType_enab ==
  data: snrType input Enum: Enum_tbm_snrType; enab_Pirelle output boolean; enab_Sansata output boolean
function [enab_Pirelle,enab_Sansata] = fcn(snrType)

enab_Pirelle = false;
enab_Sansata = false;

switch snrType
    case Enum_tbm_snrType.Pirelle
        enab_Pirelle = true;
    case Enum_tbm_snrType.Sansata  
        enab_Sansata = true;
    
end

== matlab function mVeh_fun_tbm/cu_tbm/tbm_sensor/perSnrType_selectOut ==
  data: snrType input Enum: Enum_tbm_snrType; boutFlag_4w output boolean size=4; pirelle_boutFlag_4w input boolean size=4; sansata_boutFlag_4w input boolean size=4
function boutFlag_4w  = fcn(snrType, pirelle_boutFlag_4w, sansata_boutFlag_4w)

boutFlag_4w = [false; false; false; false];

switch snrType
    case Enum_tbm_snrType.Pirelle
        boutFlag_4w = pirelle_boutFlag_4w;
    case Enum_tbm_snrType.Sansata  
        boutFlag_4w = sansata_boutFlag_4w;
    
end

== matlab function mVeh_fun_tbm/cu_tbm/asm_canMsg/to_suspension/MATLAB Function ==
  data: suspCtr_enab input boolean; suspCtr_actv_4w output boolean size=4; suspCtr_actv_4w_in input boolean size=4
function suspCtr_actv_4w = fcn(suspCtr_enab, suspCtr_actv_4w_in)

suspCtr_actv_4w = [false; false; false; false];

if suspCtr_enab
  suspCtr_actv_4w = suspCtr_actv_4w_in;  
    
end

== matlab function mVeh_fun_tbm/cu_tbm/MATLAB Function1 ==
  data: timestamp input; timestamp_sec output
function timestamp_sec = fcn(timestamp)

    timestamp_sec = single(timestamp / 1000000);
end

== matlab function mVeh_fun_tbm/cu_tbm/MATLAB Function2 ==
  data: timestamp input; timestamp_sec output
function timestamp_sec = fcn(timestamp)

    timestamp_sec = single(timestamp / 1000000);
end

== matlab function mVeh_fun_tbm/cu_tbm/Subsystem1/write VCU_14/canPack_nt2ch2_v1_1da02.dbc:VCU_14/varabToFixed_8byts ==
  data: u input uint8 size=8; y output uint8
function y = fcn(u)

fixed_size = 8;
y = uint8(zeros(fixed_size,1));

for i=1:fixed_size
    y(i) = u(i);
end

== matlab function mVeh_fun_tbm/cu_tbm/Subsystem1/send_ADC1_EPS_1AND2/canPack_nt2ch1_v1_1da02.dbc:ADC1_EPS_01/varabToFixed_8byts ==
  data: u input uint8 size=8; y output uint8
function y = fcn(u)

fixed_size = 8;
y = uint8(zeros(fixed_size,1));

for i=1:fixed_size
    y(i) = u(i);
end

== matlab function mVeh_fun_tbm/cu_tbm/Subsystem1/send_ADC1_EPS_1AND2/canPack_nt2ch1_v1_1da02.dbc:ADC1_EPS_02/varabToFixed_8byts ==
  data: u input uint8 size=8; y output uint8
function y = fcn(u)

fixed_size = 8;
y = uint8(zeros(fixed_size,1));

for i=1:fixed_size
    y(i) = u(i);
end

== matlab function mVeh_fun_tbm/cu_tbm/Subsystem1/ write TBM_02/canPack_nt2ch1_v1_4da01_fcc.dbc:TBM_02/varabToFixed_8byts ==
  data: u input uint8 size=8; y output uint8
function y = fcn(u)

fixed_size = 8;
y = uint8(zeros(fixed_size,1));

for i=1:fixed_size
    y(i) = u(i);
end

== matlab function mVeh_fun_tbm/cu_tbm/height_snr_VtoH ==
  data: snr_volt input double; height_m output double
function height_m = fcn(snr_volt)
% 0-10V analog signal, transfer to 125-625mm height signal
    k = 0.05;  % 50mm/V
    cnst = 0.125; % 125mm
    V_offset = 0.6; % offset of height sensor (Volts)
    height_m = k * (snr_volt + V_offset) + cnst;
end

== matlab function mVeh_fun_tbm/cu_tbm/Equation/MATLAB Function ==
  data: u input; y output
function y = fcn(u)

 y = 0.01 * u - 6.04;
